simulink model "Sim_begins"  (R2016b)
settings: Solver=FixedStepDiscrete  StartTime=0.0  StopTime=.04  FixedStep=.0001  RelTol=1e-3
libraries: simulink_extras x4
settings Model: Creator=Sayeed  LastModifiedBy=Sayeed

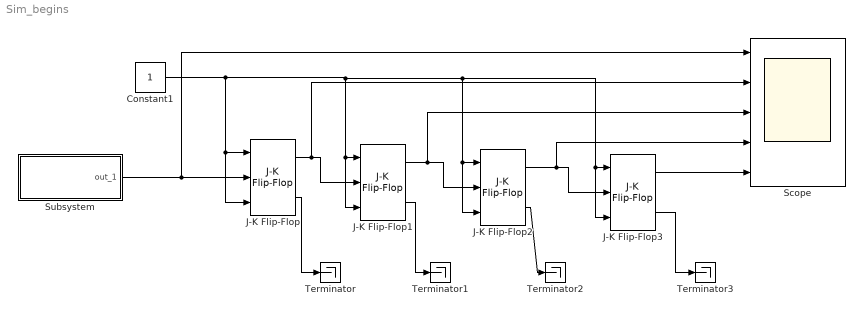
== system Sim_begins ==
  Constant1 : Constant  OutDataTypeStr=boolean
  J-K Flip-Flop{,1..3} (4 alike) : simulink_extras/Flip Flops/J-K Flip-Flop  initial_condition=0
  Scope : Scope  NumInputPorts=5
  Subsystem : Subsystem
  Terminator{,1..3} (4 alike) : Terminator
  wires:
  Constant1/1 -> J-K Flip-Flop3/3, J-K Flip-Flop3/1, J-K Flip-Flop2/3, J-K Flip-Flop2/1, J-K Flip-Flop1/3, J-K Flip-Flop1/1, J-K Flip-Flop/3, J-K Flip-Flop/1
  J-K Flip-Flop/2 -> Terminator/1
  Subsystem/1(out_1) -> Scope/1, J-K Flip-Flop/2
  J-K Flip-Flop/1 -> Scope/2, J-K Flip-Flop1/2
  J-K Flip-Flop1/1 -> Scope/3, J-K Flip-Flop2/2
  J-K Flip-Flop2/1 -> Scope/4, J-K Flip-Flop3/2
  J-K Flip-Flop1/2 -> Terminator1/1
  J-K Flip-Flop2/2 -> Terminator2/1
  J-K Flip-Flop3/2 -> Terminator3/1
  J-K Flip-Flop3/1 -> Scope/5

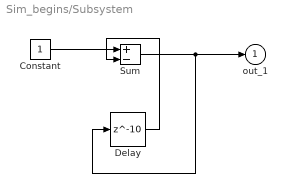
== system Sim_begins/Subsystem ==
  Constant : Constant
  Delay : Delay  DelayLength=10  InitialCondition=0
  Sum : Sum  Inputs=+-  SaturateOnIntegerOverflow=on  InputSameDT=on  OutDataTypeStr=Inherit: Same as first input
  out_1 : Outport  InitialOutput=0
  wires:
  Constant/1 -> Sum/1
  Sum/1 -> Delay/1, out_1/1
  Delay/1 -> Sum/2
